simulink model "Project_simulink"  (R2023b)
settings: Solver=VariableStepAuto  StartTime=0.0  StopTime=10.0  RelTol=1e-3
values from neighbouring files (symbols this model uses):
  a = fzero(sun_syncr, R_E)    [project.m]
  A = [A1 A2 A1 A2 A3 A3]    [project.m]
  A_0 = [-cos(phi) -sin(phi) 0; 0 0 1; -sin(phi) cos(phi) 0]    [project.m]
  A_mis_gyros = eye(3) - [0 -mis_gyros(3) mis_gyros(2); mis_gyros(3) 0 -mis_gyros(1); -mis_gyros(2) mis_gyros(1) 0]    [project.m]
  A_mis_MAG = eye(3) - [0 -mis_MAG(3) mis_MAG(2); mis_MAG(3) 0 -mis_MAG(1); -mis_MAG(2) mis_MAG(1) 0]    [project.m]
  a_S = kep_E(1)    [project.m]
  Acc = 0.75e-2    (= 0.0075)    [project.m]
  alpha = 0.9    [plotPlanet.m]    (also in project.m = [alpha_1 alpha_2]')
  alpha_error_slew_min = deg2rad(10)    [project.m]
  alpha_G_0 = deg2rad(0)    [project.m]
  Area_coil = pi * diameter_coil^2/4    (= 0.000706858347058)    [project.m]
  coil_nominal_resistance = max_voltage_torq^2/power_max_coil    (= 81.6666666667)    [project.m]
  DCM_MIS_SS = eye(3) - [0 -mis_ss(3) mis_ss(2); mis_ss(3) 0 -mis_ss(1); -mis_ss(2) mis_ss(1) 0]    [project.m]
  DCM_SS_B = eye(3)    [project.m]
  e = 0    [project.m]
  e_S = kep_E(2)    [project.m]
  f = 15    [project.m]
  f_mag = 5    [project.m]
  FS_mag = 30    [project.m]
  g = [g1_0 g2_0 g3_0 g4_0 g5_0 g6_0 g7_0 g8_0 g9_0 g10_0  g11_0  g12_0  g13_0 ... (first row only)    [IGRF13_2020.m]
  h = [h1_0 h2_0 h3_0 h4_0 h5_0 h6_0 h7_0 h8_0 h9_0 h10_0  h11_0  h12_0  h13_0 ... (first row only)    [IGRF13_2020.m]
  h_max_RW = 25    [project.m]
  I = diag([Ix_b+Ix_s,Iy_b+Iy_s,Iz_b+Iz_s])    [project.m]
  i = deg2rad(98.3)    [project.m]
  i_S = kep_E(3)    [project.m]
  Izz_RW = 1/2*m_RW*(r_RW^2)    (= 0.12168)    [project.m]
  j_b = 1.4e-3 *[0.2 0.2 1]'*m    [project.m]
  K1_slew = 433*[1,1,1]    [project.m]
  K2_slew = 2.19*[1,1,1]    [project.m]
  k_filt_g = 0.75    [project.m]
  k_filt_m = 0.75    [project.m]
  k_filt_s = 0.75    [project.m]
  K_non_lin = 0.1    [project.m]
  Kb = (1e8)    (= 100000000)    [project.m]
  Kdx = 0.5    [project.m]
  Kdy = Kdx    (= 0.5)    [project.m]
  Kdz = 0.5    [project.m]
  Kpx = 0.005    [project.m]
  Kpy = Kpx    (= 0.005)    [project.m]
  Kpz = 0.005    [project.m]
  Lin = 0.015e-2    (= 0.00015)    [project.m]
  linearity_mag_error = 0.02    [project.m]
  max_voltage_torq = 14    [project.m]
  Mounting_error_RW = eye(3) - [0 -mis_RW(3) mis_RW(2); mis_RW(3) 0 -mis_RW(1); -mis_RW(2) mis_RW(1) 0]    [project.m]
  Mounting_matrix_RW = eye(3)    [project.m]
  mu_E = astroConstants(13)    [project.m]
  n = sqrt(mu_E/a^3)    [project.m]
  N_B = [1 0 0; 0 1 0; -1 0 0; 0 -1 0; 0 0 1; 0 0 -1]'    [project.m]
  n_coil = ceil(magnetic_dipole_max/(Area_coil*current_max_coil))    [project.m]
  n_order = 13    [project.m]
  n_S = 2*pi/T_S    [project.m]
  nA_coeff = n_coil*Area_coil    [project.m]
  Noise_Mag = (12e-12)^2    (= 1.44e-22)    [project.m]
  noise_pwm = 50e-6    (= 5e-05)    [project.m]
  Noise_sun_sensor = deg2rad(Acc_ss)^2*t_ss    [project.m]
  OM = deg2rad(270)    [project.m]
  om = 0    [project.m]
  om_0 = [0.08 0.08 0.08]'    [project.m]
  om_detumbling = 4*n    [project.m]
  om_error_slew_min = 0.1*n    [project.m]
  om_target = [0,0,n]'    [project.m]
  P = Fe/c    [project.m]
  r_F = [l1/2 0 0; 0 l2/2 0; -l1/2 0 0; 0 -l2/2 0; 0 0 (l3+l3_s)/2; 0 0 -(l3+l3_s)/2]'    [project.m]
  R_th = 0.1    [project.m]
  residual_dipole = abs(0.005*magnetic_dipole_max*randn)    [project.m]
  resistance_tol = 0.05*randn    [project.m]
  rho_d = 0.1*ones(6,1)    [project.m]
  rho_S = [0.5, 0.5, 0.5, 0.5, 0.5, 0.1]    [project.m]
  RW_axis = [0;0;1]    [project.m]
  sample_time = 1/f    (= 0.0666666666667)    [project.m]
  sample_time_mag = 1/f_mag    (= 0.2)    [project.m]
  Sens = 100e-6/1e-9    (= 100000)    [project.m]
  Sensor_fov_direction = cos(FS/2)    [project.m]
  Sensor_normal_direction = [0 0 -1]'    [project.m]
  SF_a = 30 * 1e-6    (= 3e-05)    [project.m]
  SF_nl = 30 * 1e-6    (= 3e-05)    [project.m]
  SF_r = 30 * 1e-6    (= 3e-05)    [project.m]
  T_RW_max = 0.2    [project.m]
  t_ss = 1/f_ss    (= 0.2)    [project.m]
  TCR = 0.0039    [project.m]
  th0 = 0    [project.m]
  th_0_S = kep_E(6)    [project.m]
  w0_RW = w_max_RW/4    (= 91.6297857297)    [project.m]
  w_max_RW = 3500*(2*pi)/60    (= 366.519142919)    [project.m]
  w_RW_error = h_RW_error/Izz_RW    (= 0.0164365548981)    [project.m]
undefined symbols (not defined in the file or in its folder): A0, DiscIntNeverNeededParam
libraries: matrix_library x18, simulink x4, vrlib x3
(part 1 of 2)
settings Model: Creator=pietr  LastModifiedBy=dav20

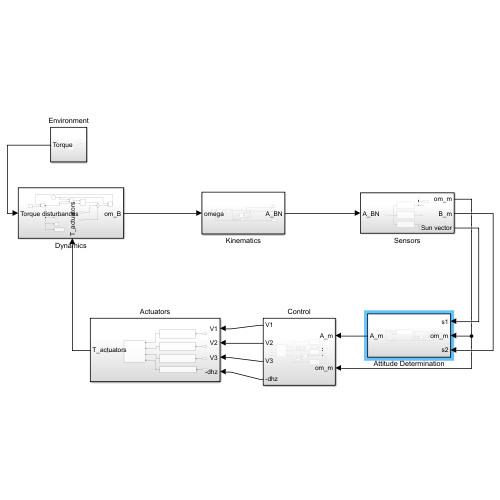
[thumbnail: Simulink's stored preview of the top-level diagram]
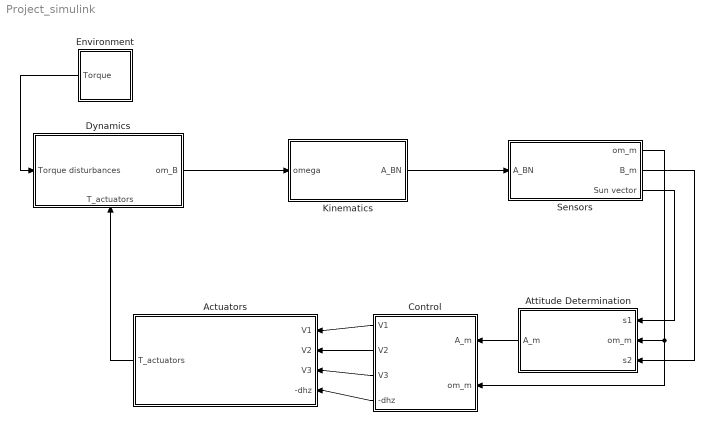
== system Project_simulink ==
  Actuators : Subsystem
  Attitude Determination : Subsystem
  Control : Subsystem
  Dynamics : Subsystem
      settings: PortSchema="{\"entries\":[{\"content\":{\"sides\":[{\"content\":{\"connectorIds\":[\"In1\"]},\"type\":\"ConnectorPlacement.EquallySpacedRectSide\",\"uuid\":\"97ef2013-c355-4554-819d-1d207ceebda7\"},{\"content\":{\"connectorIds\":[\"Out1\"],\"side\":\"RIGHT\"},\"type\":\"ConnectorPlacement.EquallySpacedRectSide\",\"uuid\":\"5691f1bb-9c80-4fa2-8587-6aaeddeffaf6\"},{\"content\":{\"side\":\"TOP\"},\"type\":\"ConnectorPlacement.EquallySpacedRectSide\",\"uuid\":\"3eac2c16-1979-435f-a318-2465fec9d9b3\"},{\"content\":{\"connectorIds\":[\"In2\"],\"side\":\"BOTTOM\"},\"type\":\"ConnectorPlacement.EquallySpacedRectSide\",\"uuid\":\"9d11ba2d-284a-4dde-a2ab-be6ae89ecb98\"}]},\"type\":\"ConnectorPlacement.EquallySpacedConnector\",\"uuid\":\"86d48b44-f40e-4c8e-8b18-c1912efaa89c\"}],\"packageUris\":[\"http://schema.mathworks.com/mf0/Connector/R2020b\"],\"version\":\"1.0\"}"
  Environment : Subsystem
  Kinematics : Subsystem
  Sensors : Subsystem
  wires:
  Control/2(V2) -> Actuators/2(V2)
  Control/3(V3) -> Actuators/3(V3)
  Control/4(-dhz) -> Actuators/4(-dhz)
  Attitude Determination/1(A_m) -> Control/1(A_m)
  Control/1(V1) -> Actuators/1(V1)
  Environment/1(Torque) -> Dynamics/1(Torque disturbances)
  Dynamics/1(om_B) -> Kinematics/1(omega)
  Kinematics/1(A_BN) -> Sensors/1(A_BN)
  Sensors/1(om_m) -> Control/2(om_m), Attitude Determination/2(om_m)
  Sensors/3(Sun vector) -> Attitude Determination/1(s1)
  Sensors/2(B_m) -> Attitude Determination/3(s2)
  Actuators/1(T_actuators) -> Dynamics/2(T_actuators)

== system Project_simulink/Actuators ==
  V1 : Inport
  V2 : Inport  Port=2
  V3 : Inport  Port=3
  -dhz : Inport  Port=4
  Magnetorquers1 : Subsystem
  Magnetorquers2 : Subsystem
  Magnetorquers3 : Subsystem
  Reaction wheel : Subsystem
  control mode torque : Subsystem
  T_actuators : Outport
  wires:
  Magnetorquers2/1(m_y) -> control mode torque/2(m_y)
  Magnetorquers1/1(m_x) -> control mode torque/1(m_x)
  Magnetorquers3/1(m_z) -> control mode torque/3(m_z)
  Reaction wheel/1(T_RW_Z) -> control mode torque/4(T_RW_Z)
  control mode torque/1(T_actuators) -> T_actuators/1
  V1/1 -> Magnetorquers1/1(Magnetorquer command [V])
  V2/1 -> Magnetorquers2/1(Magnetorquer command [V])
  V3/1 -> Magnetorquers3/1(Magnetorquer command [V])
  -dhz/1 -> Reaction wheel/1(Required derivative angular momentum)

== system Project_simulink/Attitude Determination ==
  s1 : Inport
  om_m : Inport  Port=2
  s2 : Inport  Port=3
  "Attitude determination Wabha problem " : Subsystem
  Attitude determination kinematic method : Subsystem
  Dot Product : DotProduct  OutDataTypeStr=Inherit: Inherit via internal rule
  Switch : Switch  Criteria=u2 > Threshold  Threshold=0.5  SaturateOnIntegerOverflow=off  InputSameDT=off
  A_m : Outport
  wires:
  s2/1 -> "Attitude determination Wabha problem "/2(s2)
  [S_N] -> "Attitude determination Wabha problem "/3(v1)
  [B_N] -> "Attitude determination Wabha problem "/4(v2)
  "Attitude determination Wabha problem "/1(A_m_sensor) -> Switch/1, Attitude determination kinematic method/1(A_m)
  om_m/1 -> Attitude determination kinematic method/3(omega)
  Attitude determination kinematic method/1(A_m_gyro) -> Switch/3
  Switch/1 -> A_m/1
  Dot Product/1 -> Attitude determination kinematic method/2(s1_cond), Switch/2  "sun_sensor_condition"
  s1/1 -> Dot Product/2, Dot Product/1, "Attitude determination Wabha problem "/1(s1)

== system Project_simulink/Control ==
  A_m : Inport
  om_m : Inport  Port=2
  3-axis stabilization : Subsystem
  Detumbling : Subsystem
  Flag condition : Subsystem
  Norm : Subsystem
  Slew manouevre : Subsystem
  To Workspace : ToWorkspace  VariableName=flag_det_slew  SampleTime=-1
  To Workspace1 : ToWorkspace  VariableName=flag_slew_nom  SampleTime=-1
  control mode input actuators : Subsystem
  flag_slewtonom : Subsystem
  V1 : Outport
  V2 : Outport  Port=2
  V3 : Outport  Port=3
  -dhz : Outport  Port=4
  tag scope: flag_det_slew=global, flag_slew_nom=global
  wires:
  A_m/1 -> 3-axis stabilization/2(In2), Slew manouevre/2(In2)
  3-axis stabilization/1(V_nominal) -> control mode input actuators/3(V_nominal)
  Norm/1(norm om_m) -> Flag condition/1(norm om_m)
  om_m/1 -> Norm/1(om_m), Detumbling/1(om_m), flag_slewtonom/1(om_m), 3-axis stabilization/1(om_m), Slew manouevre/1(om_m)
  Detumbling/1(V_detumb1) -> control mode input actuators/1(V_detumbling)
  Slew manouevre/1(V_slew_manouevre) -> control mode input actuators/2(V_slew)
  Slew manouevre/2(alpha errors) -> flag_slewtonom/2(alpha errors)
  flag_slewtonom/1(flag_slew_nom) -> [flag_slew_nom], To Workspace1/1
  Flag condition/1(flag) -> To Workspace/1, [flag_det_slew]
  control mode input actuators/1(V1) -> V1/1
  control mode input actuators/2(V2) -> V2/1
  control mode input actuators/3(V3) -> V3/1
  control mode input actuators/4(-dhz) -> -dhz/1

== system Project_simulink/Dynamics ==
  Torque disturbances : Inport
  T_actuators : Inport  Port=2
  Constant5 : Constant  Value=om_0
  Constant7 : Constant  Value=I
  Cross Product : matrix_library/Cross Product
  Integrator : Integrator  InitialConditionSource=external  InitialCondition=om_0
  Product : Product  Multiplication=Matrix(*)
  Product1 : Product  Inputs=/*  Multiplication=Matrix(*)
  Sum : Sum  Inputs=+++
  To Workspace2 : ToWorkspace  VariableName=om_B  SampleTime=-1
  om_B : Outport
  tag scope: om_B=global
  wires:
  Integrator/1 -> To Workspace2/1, [om_B], om_B/1, Cross Product/2, Product/2
  Product/1 -> Cross Product/1
  Constant5/1 -> Integrator/2
  Constant7/1 -> Product/1, Product1/1
  Product1/1 -> Integrator/1
  Cross Product/1 -> Sum/1
  Torque disturbances/1 -> Sum/2
  T_actuators/1 -> Sum/3
  Sum/1 -> Product1/2

== system Project_simulink/Environment ==
  Gravity Gradient Torque : Subsystem
  Magnetic Torque : Subsystem
  Orbit Definition : Subsystem
  SRP : Subsystem
  Sum : Sum
  To Workspace : ToWorkspace  VariableName=GG  SampleTime=-1
  To Workspace1 : ToWorkspace  VariableName=MAG  SampleTime=-1
  To Workspace2 : ToWorkspace  VariableName=SRP  SampleTime=-1
  To Workspace3 : ToWorkspace  VariableName=Torque  SampleTime=-1
  Torque : Outport
  tag scope: theta=global, theta_dot=global
  wires:
  Orbit Definition/3(r_direction) -> Magnetic Torque/2(r_direction)
  Orbit Definition/2(r_magnitude) -> Gravity Gradient Torque/2(r_magnitude), Magnetic Torque/1(r_magnitude)
  [A_BN] -> Magnetic Torque/3(A_BN), SRP/1(A_BN), Orbit Definition/1(A_BN)
  [A_BL] -> Gravity Gradient Torque/1(A_BL)
  Orbit Definition/1(theta) -> [theta]
  Orbit Definition/4(S_N) -> SRP/2(S_N)
  Orbit Definition/5(theta_dot) -> [theta_dot]
  SRP/1(Output1) -> To Workspace2/1
  Gravity Gradient Torque/1(Gravity Gradient Torque) -> Sum/1, To Workspace/1
  Sum/1 -> Torque/1, To Workspace3/1
  Magnetic Torque/1(Mag_Torque) -> Sum/2, To Workspace1/1

== system Project_simulink/Kinematics ==
  omega : Inport
  Antisymmetric matrix of omega : Subsystem
  Matrix A_BN : Subsystem
  Matrix A_LN : Subsystem
  Matrix Multiply : Product  Multiplication=Matrix(*)
  Product1 : Product  Multiplication=Matrix(*)
  To Workspace1 : ToWorkspace  VariableName=om_N  SampleTime=-1
  Transpose : Math  Operator=transpose
  Transpose1 : Math  Operator=transpose
  A_BN : Outport
  tag scope: A_BL=global, A_BN=global, A_LN=global
  wires:
  omega/1 -> Product1/2, Antisymmetric matrix of omega/1(omega)
  Antisymmetric matrix of omega/1(-omega^) -> Matrix A_BN/1(-omega^)
  Matrix A_BN/1(A_BN) -> A_BN/1, [A_BN], Matrix Multiply/1, Transpose1/1
  Matrix A_LN/1(A_LN) -> [A_LN], Transpose/1
  Transpose/1 -> Matrix Multiply/2
  Matrix Multiply/1 -> [A_BL]
  [theta] -> Matrix A_LN/1(theta)
  Product1/1 -> To Workspace1/1
  Transpose1/1 -> Product1/1

== system Project_simulink/Sensors ==
  A_BN : Inport
  Gyro : Subsystem
  Magnetometer : Subsystem
  Sun sensor : Subsystem
  To Workspace : ToWorkspace  VariableName=om_m  SaveFormat=Timeseries  SampleTime=-1
  To Workspace1 : ToWorkspace  VariableName=B_meas  SampleTime=-1
  om_m : Outport
  B_m : Outport  Port=2
  Sun vector : Outport  Port=3
  tag scope: B_m=global
  wires:
  Sun sensor/1(Sun vector measurement) -> Sun vector/1
  Gyro/1(om_m) -> To Workspace/1, om_m/1
  Magnetometer/1(Output) -> [B_m], To Workspace1/1, B_m/1
  A_BN/1 -> Gyro/1(A_BN), Magnetometer/1(A_BN), Sun sensor/1(A_BN)

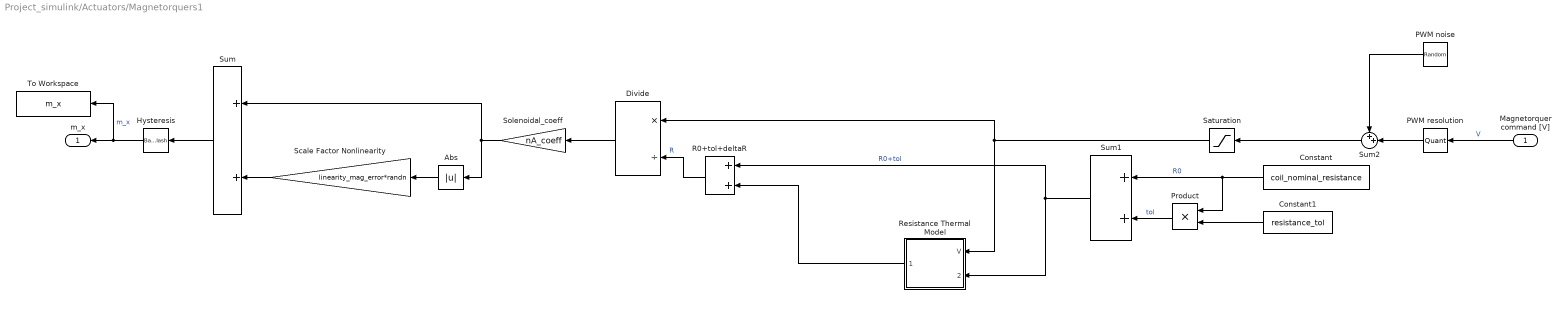
== system Project_simulink/Actuators/Magnetorquers1 ==
  Magnetorquer command [V] : Inport
  Abs : Abs  SaturateOnIntegerOverflow=off
  Constant : Constant  Value=coil_nominal_resistance
  Constant1 : Constant  Value=resistance_tol
  Divide : Product  Inputs=*/
  Hysteresis : Backlash  BacklashWidth=residual_dipole*2
  PWM noise : RandomNumber  Variance=noise_pwm^2  SampleTime=sample_time
  PWM resolution : Quantizer  QuantizationInterval=resolution_pwm
  Product : Product
  R0+tol+deltaR : Sum
  Resistance Thermal Model : Subsystem
  Saturation : Saturate  UpperLimit=max_voltage_torq  LowerLimit=-max_voltage_torq
  Scale Factor Nonlinearity : Gain  Gain=linearity_mag_error*randn
  Solenoidal_coeff : Gain  Gain=nA_coeff
  Sum : Sum
  Sum1 : Sum
  Sum2 : Sum  Inputs=++|
  To Workspace : ToWorkspace  VariableName=m_x  SampleTime=-1
  m_x : Outport
  wires:
  Sum/1 -> Hysteresis/1
  Solenoidal_coeff/1 -> Abs/1, Sum/1
  Scale Factor Nonlinearity/1 -> Sum/2
  Sum1/1 -> Resistance Thermal Model/2(R0+tol), R0+tol+deltaR/1  "R0+tol"
  Constant/1 -> Product/1, Sum1/1  "R0"
  Product/1 -> Sum1/2  "tol"
  Constant1/1 -> Product/2
  Divide/1 -> Solenoidal_coeff/1
  R0+tol+deltaR/1 -> Divide/2  "R"
  Resistance Thermal Model/1(delta R) -> R0+tol+deltaR/2
  Sum2/1 -> Saturation/1
  PWM resolution/1 -> Sum2/2
  PWM noise/1 -> Sum2/1
  Magnetorquer command [V]/1 -> PWM resolution/1  "V"
  Saturation/1 -> Resistance Thermal Model/1(V), Divide/1
  Abs/1 -> Scale Factor Nonlinearity/1
  Hysteresis/1 -> To Workspace/1, m_x/1  "m_x"

== system Project_simulink/Actuators/Magnetorquers2 ==
  Magnetorquer command [V] : Inport
  Abs : Abs  SaturateOnIntegerOverflow=off
  Constant : Constant  Value=coil_nominal_resistance
  Constant1 : Constant  Value=resistance_tol
  Divide : Product  Inputs=*/
  Hysteresis : Backlash  BacklashWidth=residual_dipole*2
  PWM noise : RandomNumber  Variance=noise_pwm^2  SampleTime=sample_time
  PWM resolution : Quantizer  QuantizationInterval=resolution_pwm
  Product : Product
  R0+tol+deltaR : Sum
  Resistance Thermal Model : Subsystem
  Saturation : Saturate  UpperLimit=max_voltage_torq  LowerLimit=-max_voltage_torq
  Scale Factor Nonlinearity : Gain  Gain=linearity_mag_error*randn
  Solenoidal_coeff : Gain  Gain=nA_coeff
  Sum : Sum
  Sum1 : Sum
  Sum2 : Sum  Inputs=++|
  To Workspace : ToWorkspace  VariableName=m_y  SampleTime=-1
  m_y : Outport
  wires:
  Abs/1 -> Scale Factor Nonlinearity/1
  Saturation/1 -> Resistance Thermal Model/1(V), Divide/1
  Magnetorquer command [V]/1 -> PWM resolution/1  "V"
  PWM noise/1 -> Sum2/1
  PWM resolution/1 -> Sum2/2
  Sum2/1 -> Saturation/1
  Resistance Thermal Model/1(delta R) -> R0+tol+deltaR/2
  R0+tol+deltaR/1 -> Divide/2  "R"
  Divide/1 -> Solenoidal_coeff/1
  Constant1/1 -> Product/2
  Product/1 -> Sum1/2  "tol"
  Constant/1 -> Sum1/1, Product/1  "R0"
  Sum1/1 -> Resistance Thermal Model/2(R0+tol), R0+tol+deltaR/1  "R0+tol"
  Scale Factor Nonlinearity/1 -> Sum/2
  Solenoidal_coeff/1 -> Abs/1, Sum/1
  Sum/1 -> Hysteresis/1
  Hysteresis/1 -> To Workspace/1, m_y/1  "m_x"

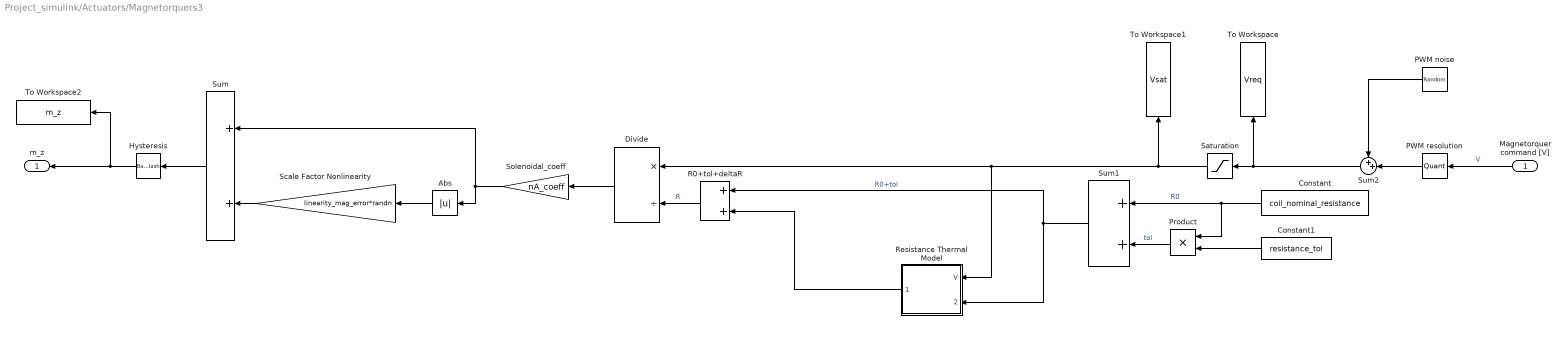
== system Project_simulink/Actuators/Magnetorquers3 ==
  Magnetorquer command [V] : Inport
  Abs : Abs  SaturateOnIntegerOverflow=off
  Constant : Constant  Value=coil_nominal_resistance
  Constant1 : Constant  Value=resistance_tol
  Divide : Product  Inputs=*/
  Hysteresis : Backlash  BacklashWidth=residual_dipole*2
  PWM noise : RandomNumber  Variance=noise_pwm^2  SampleTime=sample_time
  PWM resolution : Quantizer  QuantizationInterval=resolution_pwm
  Product : Product
  R0+tol+deltaR : Sum
  Resistance Thermal Model : Subsystem
  Saturation : Saturate  UpperLimit=max_voltage_torq  LowerLimit=-max_voltage_torq
  Scale Factor Nonlinearity : Gain  Gain=linearity_mag_error*randn
  Solenoidal_coeff : Gain  Gain=nA_coeff
  Sum : Sum
  Sum1 : Sum
  Sum2 : Sum  Inputs=++|
  To Workspace : ToWorkspace  VariableName=Vreq  SampleTime=-1
  To Workspace1 : ToWorkspace  VariableName=Vsat  SampleTime=-1
  To Workspace2 : ToWorkspace  VariableName=m_z  SampleTime=-1
  m_z : Outport
  wires:
  Abs/1 -> Scale Factor Nonlinearity/1
  Saturation/1 -> Resistance Thermal Model/1(V), Divide/1, To Workspace1/1
  Magnetorquer command [V]/1 -> PWM resolution/1  "V"
  PWM noise/1 -> Sum2/1
  PWM resolution/1 -> Sum2/2
  Sum2/1 -> Saturation/1, To Workspace/1
  Resistance Thermal Model/1(delta R) -> R0+tol+deltaR/2
  R0+tol+deltaR/1 -> Divide/2  "R"
  Divide/1 -> Solenoidal_coeff/1
  Constant1/1 -> Product/2
  Product/1 -> Sum1/2  "tol"
  Constant/1 -> Sum1/1, Product/1  "R0"
  Sum1/1 -> Resistance Thermal Model/2(R0+tol), R0+tol+deltaR/1  "R0+tol"
  Scale Factor Nonlinearity/1 -> Sum/2
  Solenoidal_coeff/1 -> Sum/1, Abs/1
  Sum/1 -> Hysteresis/1
  Hysteresis/1 -> To Workspace2/1, m_z/1

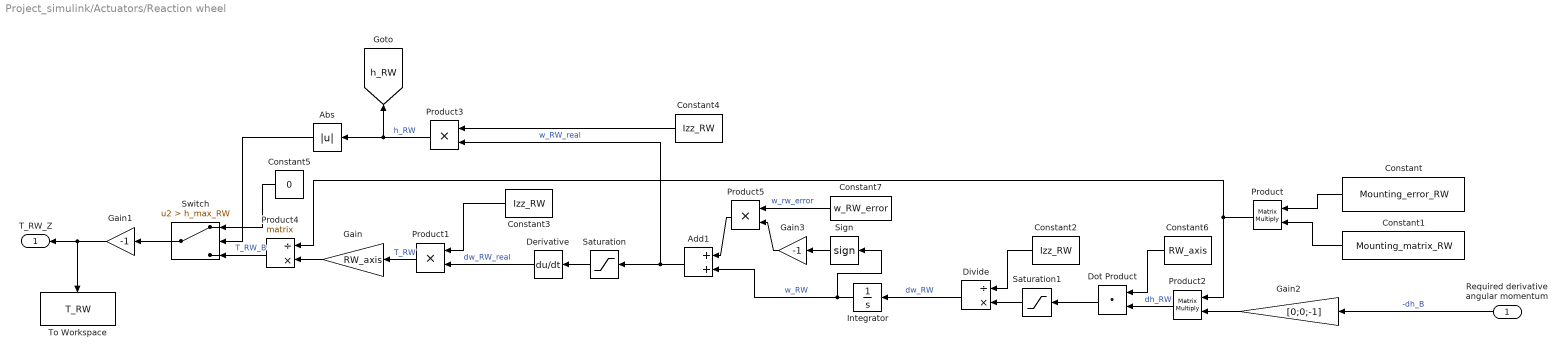
== system Project_simulink/Actuators/Reaction wheel ==
  Required derivative angular momentum : Inport
  Abs : Abs  SaturateOnIntegerOverflow=off
  Add1 : Sum
  Constant : Constant  Value=Mounting_error_RW
  Constant1 : Constant  Value=Mounting_matrix_RW
  Constant2 : Constant  Value=Izz_RW
  Constant3 : Constant  Value=Izz_RW
  Constant4 : Constant  Value=Izz_RW
  Constant5 : Constant  Value=0
  Constant6 : Constant  Value=RW_axis
  Constant7 : Constant  Value=w_RW_error
  Derivative : Derivative
  Divide : Product  Inputs=/*
  Dot Product : DotProduct  OutDataTypeStr=Inherit: Inherit via internal rule
  Gain : Gain  Gain=RW_axis
  Gain1 : Gain  Gain=-1
  Gain2 : Gain  Gain=[0;0;-1]
  Gain3 : Gain  Gain=-1
  Integrator : Integrator  InitialCondition=w0_RW
  Product : Product  Multiplication=Matrix(*)
  Product1 : Product
  Product2 : Product  Multiplication=Matrix(*)
  Product3 : Product
  Product4 : Product  Inputs=/*  Multiplication=Matrix(*)
  Product5 : Product
  Saturation : Saturate  UpperLimit=w_max_RW  LowerLimit=-w_max_RW
  Saturation1 : Saturate  UpperLimit=T_RW_max  LowerLimit=-T_RW_max
  Sign : Signum
  Switch : Switch  Criteria=u2 > Threshold  Threshold=h_max_RW  SaturateOnIntegerOverflow=off  InputSameDT=off
  To Workspace : ToWorkspace  VariableName=T_RW  SampleTime=-1
  T_RW_Z : Outport
  tag scope: h_RW=global
  wires:
  Constant/1 -> Product/1
  Constant1/1 -> Product/2
  Product/1 -> Product2/1, Product4/1
  Required derivative angular momentum/1 -> Gain2/1  "-dh_B"
  Product2/1 -> Dot Product/2  "dh_RW"
  Constant2/1 -> Divide/1
  Divide/1 -> Integrator/1  "dw_RW"
  Integrator/1 -> Sign/1, Add1/2  "w_RW"
  Add1/1 -> Product3/2, Saturation/1  "w_RW_real"
  Saturation/1 -> Derivative/1
  Saturation1/1 -> Divide/2
  Derivative/1 -> Product1/2  "dw_RW_real"
  Constant3/1 -> Product1/1
  Product1/1 -> Gain/1  "T_RW"
  Constant4/1 -> Product3/1
  Product3/1 -> Abs/1, [h_RW]  "h_RW"
  Product4/1 -> Switch/3  "T_RW_B"
  Constant5/1 -> Switch/1
  Abs/1 -> Switch/2
  Dot Product/1 -> Saturation1/1
  Constant6/1 -> Dot Product/1
  Gain/1 -> Product4/2
  Switch/1 -> Gain1/1
  Gain2/1 -> Product2/2
  Sign/1 -> Gain3/1
  Gain3/1 -> Product5/2
  Constant7/1 -> Product5/1  "w_rw_error"
  Product5/1 -> Add1/1
  Gain1/1 -> To Workspace/1, T_RW_Z/1

== system Project_simulink/Actuators/control mode torque ==
  m_x : Inport
  m_y : Inport  Port=2
  m_z : Inport  Port=3
  T_RW_Z : Inport  Port=4
  Subsystem : Subsystem
  Subsystem1 : Subsystem
  Switch : Switch  Threshold=0.5  SaturateOnIntegerOverflow=off  InputSameDT=off
  T_actuators : Outport
  wires:
  m_x/1 -> Subsystem/1(m_x), Subsystem1/1(m_x)
  m_y/1 -> Subsystem/2(m_y), Subsystem1/2(m_y)
  T_RW_Z/1 -> Subsystem/3(T_RW)
  m_z/1 -> Subsystem1/3(m_z)
  [flag_det_slew] -> Switch/2
  Subsystem1/1(T_detumbling) -> Switch/1
  Switch/1 -> T_actuators/1
  Subsystem/1(T_slewornom) -> Switch/3

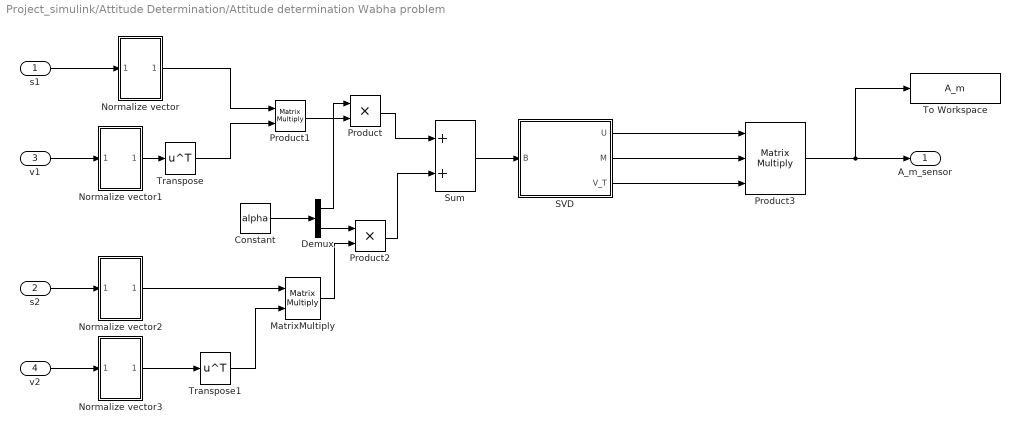
== system Project_simulink/Attitude Determination/Attitude determination Wabha problem  ==
  s1 : Inport
  s2 : Inport  Port=2
  v1 : Inport  Port=3
  v2 : Inport  Port=4
  Constant : Constant  Value=alpha
  Demux : Demux  Outputs=2
  MatrixMultiply : Product  Multiplication=Matrix(*)
  Normalize vector : Subsystem
  Normalize vector1 : Subsystem
  Normalize vector2 : Subsystem
  Normalize vector3 : Subsystem
  Product : Product
  Product1 : Product  Multiplication=Matrix(*)
  Product2 : Product
  Product3 : Product  Inputs=3  Multiplication=Matrix(*)
  SVD : MATLAB Function  TreatAsAtomicUnit=on
  Sum : Sum
  To Workspace : ToWorkspace  VariableName=A_m  SampleTime=-1
  Transpose : Math  Operator=transpose
  Transpose1 : Math  Operator=transpose
  A_m_sensor : Outport
  wires:
  Constant/1 -> Demux/1
  v1/1 -> Normalize vector1/1(In1)
  v2/1 -> Normalize vector3/1(In1)
  Transpose/1 -> Product1/2
  Product1/1 -> Product/2
  Demux/1 -> Product/1
  Transpose1/1 -> MatrixMultiply/2
  s2/1 -> Normalize vector2/1(In1)
  MatrixMultiply/1 -> Product2/2
  Demux/2 -> Product2/1
  Product2/1 -> Sum/2
  Product/1 -> Sum/1
  Sum/1 -> SVD/1(B)
  SVD/1(U) -> Product3/1
  SVD/2(M) -> Product3/2
  SVD/3(V_T) -> Product3/3
  Normalize vector1/1(Out1) -> Transpose/1
  Normalize vector2/1(Out1) -> MatrixMultiply/1
  Normalize vector3/1(Out1) -> Transpose1/1
  Product3/1 -> A_m_sensor/1, To Workspace/1
  s1/1 -> Normalize vector/1(In1)
  Normalize vector/1(Out1) -> Product1/1

== system Project_simulink/Attitude Determination/Attitude determination kinematic method ==
  A_m : Inport
  s1_cond : Inport  Port=2
  omega : Inport  Port=3
  Antisymmetric matrix of omega : Subsystem
  Matrix A_BN : Subsystem
  A_m_gyro : Outport
  wires:
  omega/1 -> Antisymmetric matrix of omega/1(omega)
  Antisymmetric matrix of omega/1(-omega^) -> Matrix A_BN/2(-omega^)
  Matrix A_BN/1(A_m_gyro) -> A_m_gyro/1
  A_m/1 -> Matrix A_BN/3(A_m)
  s1_cond/1 -> Matrix A_BN/1(s1_cond)

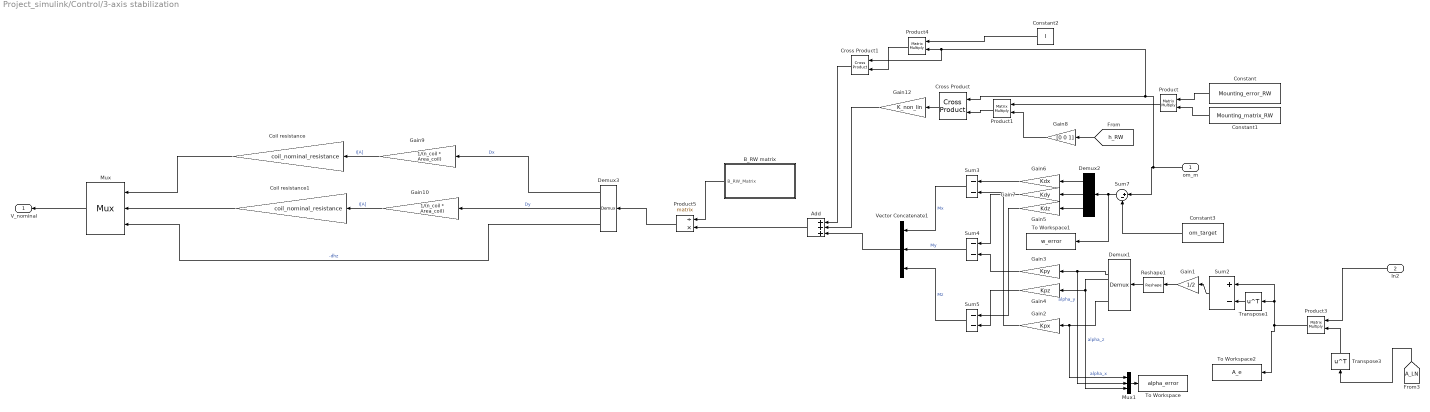
== system Project_simulink/Control/3-axis stabilization ==
  om_m : Inport
  In2 : Inport  Port=2
  Add : Sum  Inputs=+++
  B_RW matrix : Subsystem
  Coil resistance : Gain  Gain=coil_nominal_resistance
  Coil resistance1 : Gain  Gain=coil_nominal_resistance
  Constant : Constant  Value=Mounting_error_RW
  Constant1 : Constant  Value=Mounting_matrix_RW
  Constant2 : Constant  Value=I
  Constant3 : Constant  Value=om_target
  Cross Product : matrix_library/Cross Product
  Cross Product1 : vrlib/Utilities/Cross Product
  Demux1 : Demux  Outputs=9
  Demux2 : Demux  Outputs=3
  Demux3 : Demux  Outputs=3
  Gain1 : Gain  Gain=1/2
  Gain10 : Gain  Gain=1/(n_coil * Area_coil)
  Gain12 : Gain  Gain=K_non_lin
  Gain2 : Gain  Gain=Kpx
  Gain3 : Gain  Gain=Kpy
  Gain4 : Gain  Gain=Kpz
  Gain5 : Gain  Gain=Kdz
  Gain6 : Gain  Gain=Kdx
  Gain7 : Gain  Gain=Kdy
  Gain8 : Gain  Gain=[0 0 1]
  Gain9 : Gain  Gain=1/(n_coil * Area_coil)
  Mux : Mux  Inputs=3
  Mux1 : Mux  Inputs=3
  Product{,1,3..4} (4 alike) : Product  Multiplication=Matrix(*)
  Product5 : Product  Inputs=/*  Multiplication=Matrix(*)
  Reshape1 : Reshape
  Sum2 : Sum  Inputs=+-
  Sum3 : Sum  Inputs=--
  Sum4 : Sum  Inputs=--
  Sum5 : Sum  Inputs=--
  Sum7 : Sum  Inputs=|+-
  To Workspace : ToWorkspace  VariableName=alpha_error  SampleTime=-1
  To Workspace1 : ToWorkspace  VariableName=w_error  SampleTime=-1
  To Workspace2 : ToWorkspace  VariableName=A_e  SampleTime=-1
  Transpose1 : Math  Operator=transpose
  Transpose3 : Math  Operator=transpose
  Vector Concatenate1 : Concatenate  NumInputs=3
  V_nominal : Outport
  wires:
  Sum5/1 -> Vector Concatenate1/3  "Mz"
  om_m/1 -> Sum7/1, Cross Product1/1, Product4/2, Cross Product/1
  Gain2/1 -> Sum3/2
  Gain6/1 -> Sum3/1
  Demux3/2 -> Gain10/1  "Dy"
  Demux1/4 -> Mux1/3, Gain4/1  "alpha_z"
  Demux2/1 -> Gain6/1
  Gain1/1 -> Reshape1/1
  Constant3/1 -> Sum7/2
  Gain3/1 -> Sum4/2
  Product3/1 -> To Workspace2/1, Transpose1/1, Sum2/1
  Demux3/3 -> Mux/3  "-dhz"
  Demux2/3 -> Gain5/1
  Demux1/8 -> Mux1/1, Gain2/1  "alpha_x"
  Sum4/1 -> Vector Concatenate1/2  "My"
  Gain5/1 -> Sum5/1
  Gain10/1 -> Coil resistance1/1  "I[A]"
  Sum7/1 -> To Workspace1/1, Demux2/1
  B_RW matrix/1(B_RW_Matrix) -> Product5/1
  Sum2/1 -> Gain1/1
  Add/1 -> Product5/2
  Sum3/1 -> Vector Concatenate1/1  "Mx"
  Demux1/3 -> Mux1/2, Gain3/1  "alpha_y"
  Demux2/2 -> Gain7/1
  [A_LN] -> Transpose3/1
  Product4/1 -> Cross Product1/2
  Product5/1 -> Demux3/1
  Transpose1/1 -> Sum2/2
  Gain7/1 -> Sum4/1
  Reshape1/1 -> Demux1/1
  Constant2/1 -> Product4/1
  Gain9/1 -> Coil resistance/1  "I[A]"
  Transpose3/1 -> Product3/2
  Gain4/1 -> Sum5/2
  In2/1 -> Product3/1
  Coil resistance/1 -> Mux/1
  Coil resistance1/1 -> Mux/2
  Mux/1 -> V_nominal/1
  Constant/1 -> Product/1
  Constant1/1 -> Product/2
  Product/1 -> Product1/1
  [h_RW] -> Gain8/1
  Vector Concatenate1/1 -> Add/3
  Gain8/1 -> Product1/2
  Cross Product1/1 -> Add/1
  Gain12/1 -> Add/2
  Product1/1 -> Cross Product/2
  Cross Product/1 -> Gain12/1
  Demux3/1 -> Gain9/1  "Dx"
  Mux1/1 -> To Workspace/1

== system Project_simulink/Control/Detumbling ==
  om_m : Inport
  Antisymmetric matrix of omega : Subsystem
  Coil resistance2 : Gain  Gain=coil_nominal_resistance
  Coil resistance3 : Gain  Gain=coil_nominal_resistance
  Coil resistance4 : Gain  Gain=coil_nominal_resistance
  Constant : Constant  Value=Kb
  Demux4 : Demux  Outputs=3
  Gain12 : Gain  Gain=1/(n_coil * Area_coil)
  Gain13 : Gain  Gain=1/(n_coil * Area_coil)
  Gain14 : Gain  Gain=1/(n_coil * Area_coil)
  MatrixMultiply : Product  Multiplication=Matrix(*)
  Mux : Mux  Inputs=3
  Product10 : Product  Inputs=**
  Scope2 : Scope
  To Workspace : ToWorkspace  VariableName=D_desired  SampleTime=-1
  To Workspace1 : ToWorkspace  VariableName=Kb  SampleTime=-1
  V_detumb1 : Outport
  wires:
  Coil resistance4/1 -> Mux/3
  Antisymmetric matrix of omega/1(-omega^) -> MatrixMultiply/1
  Demux4/1 -> Gain14/1  "Dx"
  Demux4/3 -> Gain13/1  "Dz"
  Gain14/1 -> Coil resistance2/1  "I[A]"
  Coil resistance3/1 -> Mux/2
  om_m/1 -> Antisymmetric matrix of omega/1(omega)
  [B_m] -> MatrixMultiply/2
  Gain12/1 -> Coil resistance3/1  "I[A]"
  Gain13/1 -> Coil resistance4/1  "I[A]"
  Demux4/2 -> Gain12/1  "Dy"
  Coil resistance2/1 -> Mux/1
  MatrixMultiply/1 -> Product10/1  "dB"
  Product10/1 -> To Workspace/1, Demux4/1, Scope2/1
  Constant/1 -> Product10/2
  Mux/1 -> V_detumb1/1

== system Project_simulink/Control/Flag condition ==
  norm om_m : Inport
  Clock : Clock
  Constant2 : Constant
  Constant3 : Constant
  Constant4 : Constant  Value=0
  Delay : Delay  DelayLength=1
  Product3 : Product
  Switch : Switch  Criteria=u2 > Threshold  Threshold=om_detumbling  SaturateOnIntegerOverflow=off  InputSameDT=off
  Switch1 : Switch  Threshold=1/f  SaturateOnIntegerOverflow=off  InputSameDT=off
  flag : Outport
  wires:
  Delay/1 -> Switch1/1
  Product3/1 -> flag/1, Delay/1
  Switch1/1 -> Product3/2
  Constant2/1 -> Switch1/3
  Clock/1 -> Switch1/2
  Switch/1 -> Product3/1
  Constant4/1 -> Switch/3
  norm om_m/1 -> Switch/2
  Constant3/1 -> Switch/1

== system Project_simulink/Control/Norm ==
  om_m : Inport
  Dot Product : DotProduct  OutDataTypeStr=Inherit: Inherit via internal rule
  Square Root : Sqrt
  norm om_m : Outport
  wires:
  Square Root/1 -> norm om_m/1
  Dot Product/1 -> Square Root/1
  om_m/1 -> Dot Product/1, Dot Product/2

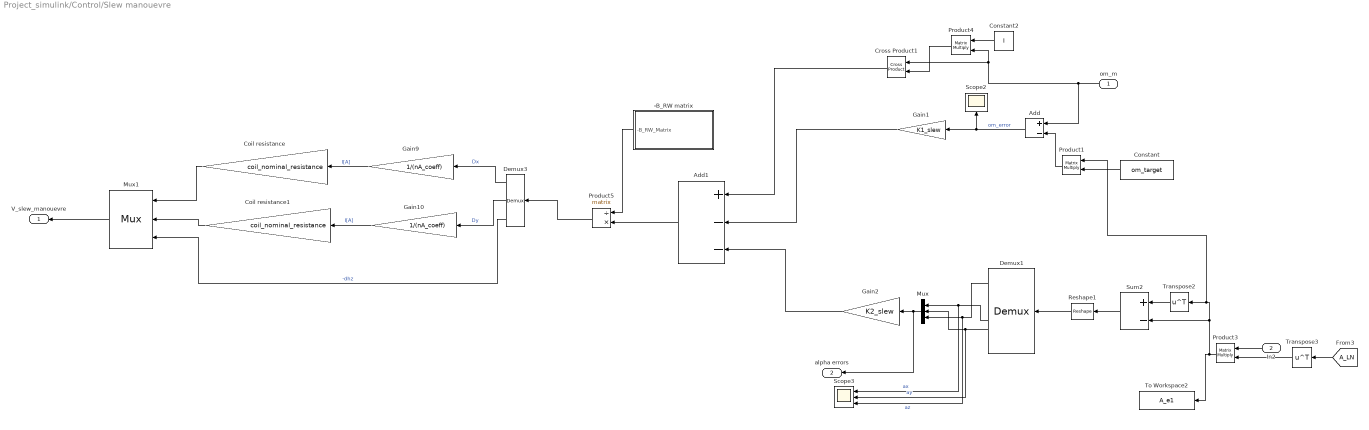
== system Project_simulink/Control/Slew manouevre ==
  om_m : Inport
  In2 : Inport  Port=2
  -B_RW matrix : Subsystem
  Add : Sum  Inputs=+-
  Add1 : Sum  Inputs=+--
  Coil resistance : Gain  Gain=coil_nominal_resistance
  Coil resistance1 : Gain  Gain=coil_nominal_resistance
  Constant : Constant  Value=om_target
  Constant2 : Constant  Value=I
  Cross Product1 : vrlib/Utilities/Cross Product
  Demux1 : Demux  Outputs=9
  Demux3 : Demux  Outputs=3
  Gain1 : Gain  Gain=K1_slew
  Gain10 : Gain  Gain=1/(nA_coeff)
  Gain2 : Gain  Gain=K2_slew
  Gain9 : Gain  Gain=1/(nA_coeff)
  Mux : Mux  Inputs=3
  Mux1 : Mux  Inputs=3
  Product1 : Product  Multiplication=Matrix(*)
  Product3 : Product  Multiplication=Matrix(*)
  Product4 : Product  Multiplication=Matrix(*)
  Product5 : Product  Inputs=/*  Multiplication=Matrix(*)
  Reshape1 : Reshape
  Scope2 : Scope
  Scope3 : Scope  NumInputPorts=3
  Sum2 : Sum  Inputs=+-
  To Workspace2 : ToWorkspace  VariableName=A_e1  SampleTime=-1
  Transpose2 : Math  Operator=transpose
  Transpose3 : Math  Operator=transpose
  V_slew_manouevre : Outport
  alpha errors : Outport  Port=2
  wires:
  Gain1/1 -> Add1/2
  Mux/1 -> alpha errors/1, Gain2/1
  In2/1 -> Product3/1
  Transpose3/1 -> Product3/2
  [A_LN] -> Transpose3/1
  Sum2/1 -> Reshape1/1
  Reshape1/1 -> Demux1/1
  Constant2/1 -> Product4/1
  Product4/1 -> Cross Product1/2
  om_m/1 -> Add/1, Product4/2, Cross Product1/1
  Cross Product1/1 -> Add1/1
  Add/1 -> Scope2/1, Gain1/1  "om_error"
  Gain2/1 -> Add1/3
  Gain9/1 -> Coil resistance/1  "I[A]"
  Coil resistance1/1 -> Mux1/2
  Demux3/1 -> Gain9/1  "Dx"
  -B_RW matrix/1(-B_RW_Matrix) -> Product5/1
  Coil resistance/1 -> Mux1/1
  Product5/1 -> Demux3/1
  Gain10/1 -> Coil resistance1/1  "I[A]"
  Add1/1 -> Product5/2
  Demux3/3 -> Mux1/3  "-dhz"
  Mux1/1 -> V_slew_manouevre/1
  Demux3/2 -> Gain10/1  "Dy"
  Product3/1 -> Sum2/2, Product1/1, Transpose2/1, To Workspace2/1
  Transpose2/1 -> Sum2/1
  Demux1/2 -> Scope3/3, Mux/3  "az"
  Demux1/6 -> Scope3/1, Mux/1  "ax"
  Demux1/7 -> Scope3/2, Mux/2  "ay"
  Constant/1 -> Product1/2
  Product1/1 -> Add/2

== system Project_simulink/Control/control mode input actuators ==
  V_detumbling : Inport
  V_slew : Inport  Port=2
  V_nominal : Inport  Port=3
  Constant : Constant  Value=0
  Demux1 : Demux  Outputs=3
  Switch{1..4} (4 alike) : Switch  Threshold=0.5  SaturateOnIntegerOverflow=off  InputSameDT=off
  V1 : Outport
  V2 : Outport  Port=2
  V3 : Outport  Port=3
  -dhz : Outport  Port=4
  wires:
  Switch2/1 -> Demux1/1
  [flag_det_slew] -> Switch4/2, Switch3/2, Switch2/2
  Demux1/3 -> Switch4/3, Switch3/1
  [flag_slew_nom] -> Switch1/2
  V_nominal/1 -> Switch1/3
  Constant/1 -> Switch3/3, Switch4/1
  V_detumbling/1 -> Switch2/1
  V_slew/1 -> Switch1/1
  Switch1/1 -> Switch2/3
  Demux1/2 -> V2/1
  Demux1/1 -> V1/1
  Switch4/1 -> -dhz/1
  Switch3/1 -> V3/1

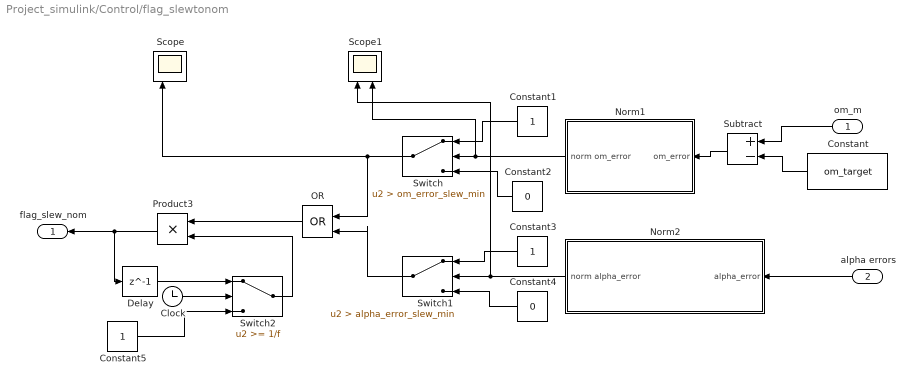
== system Project_simulink/Control/flag_slewtonom ==
  om_m : Inport
  alpha errors : Inport  Port=2
  Clock : Clock
  Constant : Constant  Value=om_target
  Constant1 : Constant
  Constant2 : Constant  Value=0
  Constant3 : Constant
  Constant4 : Constant  Value=0
  Constant5 : Constant
  Delay : Delay  DelayLength=1
  Norm1 : Subsystem
  Norm2 : Subsystem
  OR : Logic  Operator=OR  IconShape=distinctive  AllPortsSameDT=off  OutDataTypeStr=boolean
  Product3 : Product
  Scope : Scope  NumInputPorts=2
  Scope1 : Scope  NumInputPorts=2
  Subtract : Sum  Inputs=+-
  Switch : Switch  Criteria=u2 > Threshold  Threshold=om_error_slew_min  SaturateOnIntegerOverflow=off  InputSameDT=off
  Switch1 : Switch  Criteria=u2 > Threshold  Threshold=alpha_error_slew_min  SaturateOnIntegerOverflow=off  InputSameDT=off
  Switch2 : Switch  Threshold=1/f  SaturateOnIntegerOverflow=off  InputSameDT=off
  flag_slew_nom : Outport
  wires:
  Constant/1 -> Subtract/2
  Norm1/1(norm om_error) -> Scope1/2, Switch/2
  Subtract/1 -> Norm1/1(om_error)
  om_m/1 -> Subtract/1
  alpha errors/1 -> Norm2/1(alpha_error)
  Constant1/1 -> Switch/1
  Constant2/1 -> Switch/3
  Constant4/1 -> Switch1/3
  Constant3/1 -> Switch1/1
  Norm2/1(norm alpha_error) -> Scope1/1, Switch1/2
  Switch/1 -> Scope/1, OR/1
  Product3/1 -> flag_slew_nom/1, Delay/1
  OR/1 -> Product3/1
  Constant5/1 -> Switch2/3
  Clock/1 -> Switch2/2
  Delay/1 -> Switch2/1
  Switch2/1 -> Product3/2
  Switch1/1 -> OR/2

== system Project_simulink/Environment/Gravity Gradient Torque ==
  A_BL : Inport
  r_magnitude : Inport  Port=2
  Constant : Constant  Value=3
  Constant2 : Constant  Value=[1;0;0]
  Constant3 : Constant  Value=I  VectorParams1D=off
  Cross Product : matrix_library/Cross Product
  Divide : Product  Inputs=*/
  Gain : Gain  Gain=3*mu_E
  Gain1 : Gain  Gain=-1
  Matrix Multiply1 : Product  Multiplication=Matrix(*)
  Matrix Multiply2 : Product  Multiplication=Matrix(*)
  Power : Math  Operator=pow
  Gravity Gradient Torque : Outport
  wires:
  Constant3/1 -> Matrix Multiply2/1
  Matrix Multiply1/1 -> Cross Product/2, Matrix Multiply2/2  "[c1; c2; c3]"
  Cross Product/1 -> Gain/1
  Matrix Multiply2/1 -> Cross Product/1
  Constant2/1 -> Matrix Multiply1/2
  A_BL/1 -> Matrix Multiply1/1
  r_magnitude/1 -> Power/1
  Constant/1 -> Power/2
  Power/1 -> Divide/2
  Divide/1 -> Gain1/1
  Gain/1 -> Divide/1
  Gain1/1 -> Gravity Gradient Torque/1

== system Project_simulink/Environment/Magnetic Torque ==
  r_magnitude : Inport
  r_direction : Inport  Port=2
  A_BN : Inport  Port=3
  Clock : Clock
  Constant5 : Constant  Value=j_b
  Constant6 : Constant  Value=g
  Constant7 : Constant  Value=h
  Constant8 : Constant  Value=alpha_G_0
  Constant9 : Constant  Value=n_order
  Cross Product1 : matrix_library/Cross Product
  MATLAB Function : MATLAB Function  TreatAsAtomicUnit=on
  MatrixMultiply : Product  Multiplication=Matrix(*)
  Product3 : Product
  Reshape : Reshape
  Mag_Torque : Outport
  tag scope: B_B=global, B_N=global
  wires:
  Constant8/1 -> MATLAB Function/5(alpha_G_0)
  Constant6/1 -> MATLAB Function/3(g)
  Constant9/1 -> MATLAB Function/6(n_order)
  A_BN/1 -> MatrixMultiply/1
  r_magnitude/1 -> Product3/2
  Constant5/1 -> Cross Product1/1
  MatrixMultiply/1 -> [B_B], Cross Product1/2
  Cross Product1/1 -> Mag_Torque/1
  r_direction/1 -> Product3/1
  Product3/1 -> MATLAB Function/1(r_n)
  Constant7/1 -> MATLAB Function/4(h)
  Clock/1 -> MATLAB Function/2(t)
  MATLAB Function/1(B_N) -> Reshape/1
  Reshape/1 -> MatrixMultiply/2, [B_N]

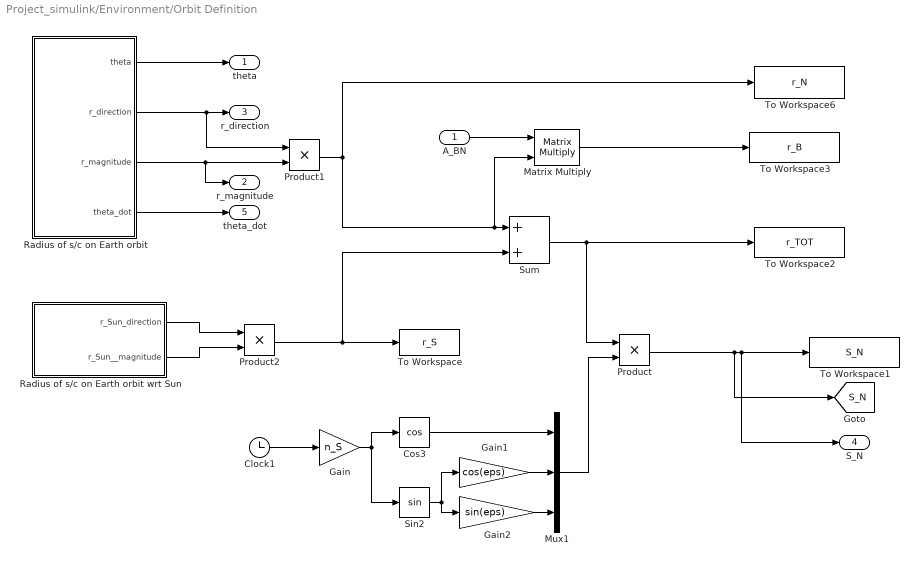
== system Project_simulink/Environment/Orbit Definition ==
  A_BN : Inport
  Clock1 : Clock
  Cos3 : Trigonometry  Operator=cos
  Gain : Gain  Gain=n_S
  Gain1 : Gain  Gain=cos(eps)
  Gain2 : Gain  Gain=sin(eps)
  Matrix Multiply : Product  Multiplication=Matrix(*)
  Mux1 : Mux  Inputs=3
  Product : Product
  Product1 : Product
  Product2 : Product
  Radius of s/c on Earth orbit : Subsystem
  Radius of s/c on Earth orbit wrt Sun : Subsystem
  Sin2 : Trigonometry
  Sum : Sum
  To Workspace : ToWorkspace  VariableName=r_S  SampleTime=-1
  To Workspace1 : ToWorkspace  VariableName=S_N  SampleTime=-1
  To Workspace2 : ToWorkspace  VariableName=r_TOT  SaveFormat=Timeseries  SampleTime=-1
  To Workspace3 : ToWorkspace  VariableName=r_B  SampleTime=-1
  To Workspace6 : ToWorkspace  VariableName=r_N  SampleTime=-1
  theta : Outport
  r_magnitude : Outport  Port=2
  r_direction : Outport  Port=3
  S_N : Outport  Port=4
  theta_dot : Outport  Port=5
  tag scope: S_N=global
  wires:
  Radius of s/c on Earth orbit/1(theta) -> theta/1
  Clock1/1 -> Gain/1
  Sum/1 -> To Workspace2/1, Product/1
  Mux1/1 -> Product/2
  Radius of s/c on Earth orbit/2(r_direction) -> Product1/1, r_direction/1
  Radius of s/c on Earth orbit/3(r_magnitude) -> r_magnitude/1, Product1/2
  Product1/1 -> To Workspace6/1, Matrix Multiply/2, Sum/1
  Radius of s/c on Earth orbit wrt Sun/2(r_Sun__magnitude) -> Product2/2
  Radius of s/c on Earth orbit wrt Sun/1(r_Sun_direction) -> Product2/1
  Product2/1 -> To Workspace/1, Sum/2
  Cos3/1 -> Mux1/1
  Gain/1 -> Sin2/1, Cos3/1
  Sin2/1 -> Gain2/1, Gain1/1
  Gain1/1 -> Mux1/2
  A_BN/1 -> Matrix Multiply/1
  Matrix Multiply/1 -> To Workspace3/1
  Radius of s/c on Earth orbit/4(theta_dot) -> theta_dot/1
  Product/1 -> S_N/1, To Workspace1/1, [S_N]
  Gain2/1 -> Mux1/3

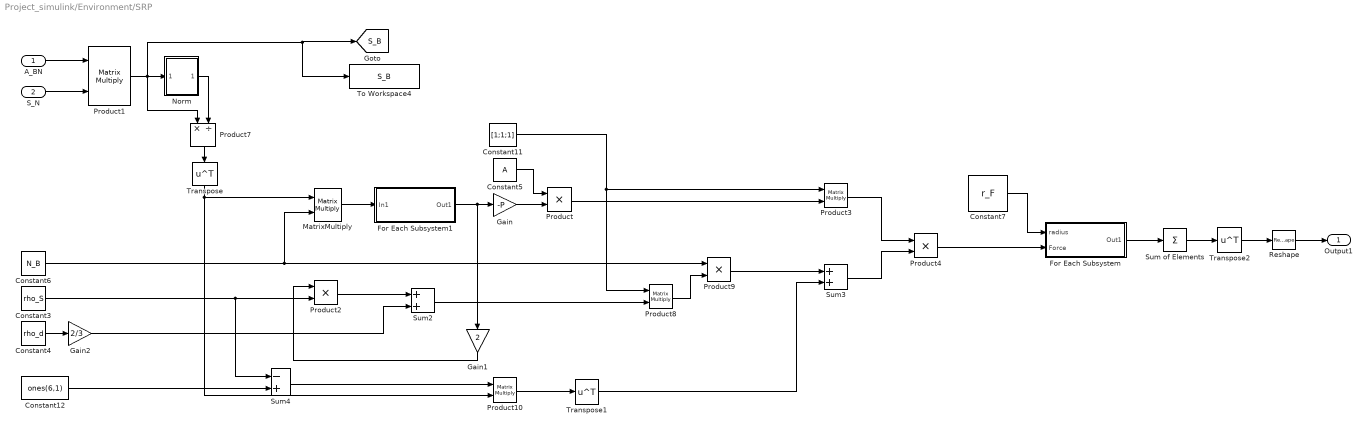
== system Project_simulink/Environment/SRP ==
  A_BN : Inport
  S_N : Inport  Port=2
  Constant11 : Constant  Value=[1;1;1]
  Constant12 : Constant  Value=ones(6,1)
  Constant3 : Constant  Value=rho_S
  Constant4 : Constant  Value=rho_d
  Constant5 : Constant  Value=A
  Constant6 : Constant  Value=N_B
  Constant7 : Constant  Value=r_F
  For Each Subsystem : Subsystem  TreatAsAtomicUnit=on
  For Each Subsystem1 : Subsystem  TreatAsAtomicUnit=on
  Gain : Gain  Gain=-P
  Gain1 : Gain  Gain=2
  Gain2 : Gain  Gain=2/3
  MatrixMultiply : Product  Multiplication=Matrix(*)
  Norm : Subsystem
  Product{,2,4,9} (4 alike) : Product
  Product{1,3,8,10} (4 alike) : Product  Multiplication=Matrix(*)
  Product7 : Product  Inputs=*/
  Reshape : Reshape
  Sum of Elements : Sum  Inputs=+  CollapseMode=Specified dimension  CollapseDim=2
  Sum2 : Sum
  Sum3 : Sum
  Sum4 : Sum  Inputs=-+
  To Workspace4 : ToWorkspace  VariableName=S_B  SampleTime=-1
  Transpose : Math  Operator=transpose
  Transpose1 : Math  Operator=transpose
  Transpose2 : Math  Operator=transpose
  Output1 : Outport
  tag scope: S_B=global
  wires:
  Norm/1(Out1) -> Product7/2
  Product2/1 -> Sum2/1
  Product7/1 -> Transpose/1
  Product1/1 -> [S_B], To Workspace4/1, Norm/1(In1), Product7/1
  Constant4/1 -> Gain2/1
  MatrixMultiply/1 -> For Each Subsystem1/1(In1)
  Sum4/1 -> Product10/1
  Gain/1 -> Product/2
  Constant6/1 -> Product9/1, MatrixMultiply/2
  Gain2/1 -> Sum2/2
  Constant3/1 -> Sum4/1, Product2/2
  Sum of Elements/1 -> Transpose2/1
  Product10/1 -> Transpose1/1
  Product4/1 -> For Each Subsystem/2(Force)
  Gain1/1 -> Product2/1
  Product3/1 -> Product4/1
  Product9/1 -> Sum3/1
  Transpose1/1 -> Sum3/2
  Product8/1 -> Product9/2
  Constant5/1 -> Product/1
  Sum2/1 -> Product8/2
  Transpose/1 -> Product10/2, MatrixMultiply/1
  A_BN/1 -> Product1/1
  Transpose2/1 -> Reshape/1
  Constant7/1 -> For Each Subsystem/1(radius)
  Constant11/1 -> Product8/1, Product3/1
  Product/1 -> Product3/2
  For Each Subsystem/1(Out1) -> Sum of Elements/1
  S_N/1 -> Product1/2
  For Each Subsystem1/1(Out1) -> Gain1/1, Gain/1
  Sum3/1 -> Product4/2
  Reshape/1 -> Output1/1
  Constant12/1 -> Sum4/2

== system Project_simulink/Kinematics/Antisymmetric matrix of omega ==
  omega : Inport
  Constant1 : Constant  Value=[1; 0; 0]  VectorParams1D=off
  Constant2 : Constant  Value=[0; 1; 0]
  Constant3 : Constant  Value=[0; 0; 1]
  Cross Product : matrix_library/Cross Product
  Cross Product1 : matrix_library/Cross Product
  Cross Product2 : matrix_library/Cross Product
  Gain : Gain  Gain=-1
  Mux : Mux  Inputs=3
  Reshape : Reshape  OutputDimensionality=Customize  OutputDimensions=[3,3]
  -omega^ : Outport
  wires:
  omega/1 -> Cross Product/1, Cross Product1/1, Cross Product2/1
  Constant3/1 -> Cross Product2/2
  Cross Product2/1 -> Mux/3
  Cross Product1/1 -> Mux/2
  Mux/1 -> Reshape/1
  Constant2/1 -> Cross Product1/2
  Constant1/1 -> Cross Product/2
  Cross Product/1 -> Mux/1
  Reshape/1 -> Gain/1
  Gain/1 -> -omega^/1

== system Project_simulink/Kinematics/Matrix A_BN ==
  -omega^ : Inport
  Constant5 : Constant  Value=A_0
  Integrator : Integrator  InitialConditionSource=external  InitialCondition=A0
  Orthonormalization of A(t) : Subsystem
  Product : Product  Multiplication=Matrix(*)
  To Workspace : ToWorkspace  VariableName=A_BN  SampleTime=-1
  To Workspace1 : ToWorkspace  VariableName=omega_mat  SampleTime=-1
  A_BN : Outport
  wires:
  Constant5/1 -> Integrator/2
  Orthonormalization of A(t)/1(A(t) orthonormal) -> To Workspace/1, A_BN/1, Product/2  "A_BN"
  Integrator/1 -> Orthonormalization of A(t)/1(A(t))  "A(t)"
  Product/1 -> Integrator/1
  -omega^/1 -> To Workspace1/1, Product/1

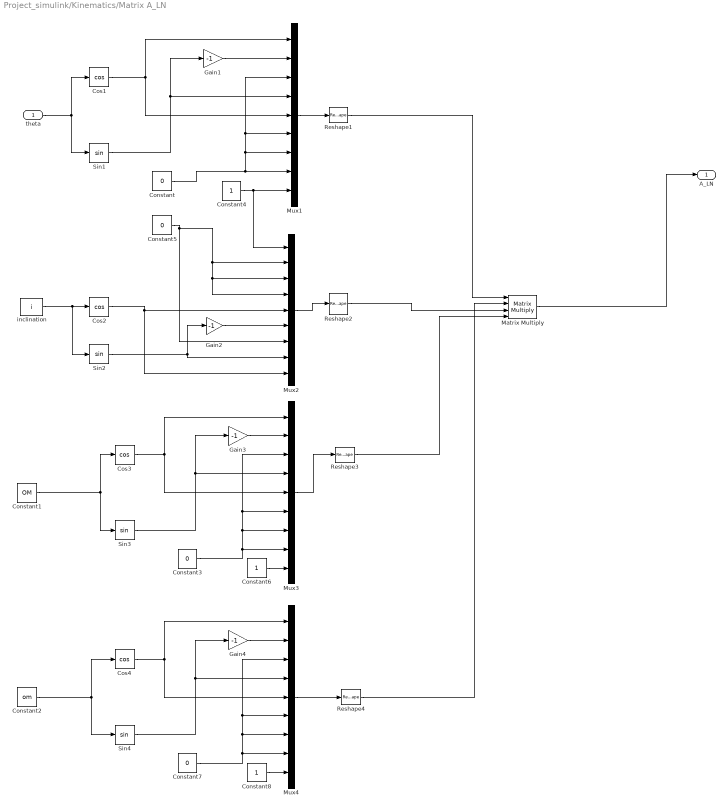
== system Project_simulink/Kinematics/Matrix A_LN ==
  theta : Inport
  Constant{,3,5,7} (4 alike) : Constant  Value=0
  Constant1 : Constant  Value=OM
  Constant2 : Constant  Value=om
  Constant4 : Constant
  Constant6 : Constant
  Constant8 : Constant
  Cos{1..4} (4 alike) : Trigonometry  Operator=cos
  Gain{1..4} (4 alike) : Gain  Gain=-1
  Matrix Multiply : Product  Inputs=4  Multiplication=Matrix(*)
  Mux{1..4} (4 alike) : Mux  Inputs=9
  Reshape{1..4} (4 alike) : Reshape  OutputDimensionality=Customize  OutputDimensions=[3,3]
  Sin{1..4} (4 alike) : Trigonometry
  inclination : Constant  Value=i
  A_LN : Outport
  wires:
  Constant5/1 -> Mux2/4, Mux2/3, Mux2/2, Mux2/7
  Gain2/1 -> Mux2/6
  Constant4/1 -> Mux2/1, Mux1/9
  Sin2/1 -> Gain2/1, Mux2/8
  Cos2/1 -> Mux2/5, Mux2/9
  Gain1/1 -> Mux1/2
  Sin1/1 -> Gain1/1, Mux1/4
  theta/1 -> Cos1/1, Sin1/1
  Constant/1 -> Mux1/8, Mux1/7, Mux1/6, Mux1/3
  Mux2/1 -> Reshape2/1
  inclination/1 -> Sin2/1, Cos2/1
  Mux1/1 -> Reshape1/1
  Cos1/1 -> Mux1/5, Mux1/1
  Cos3/1 -> Mux3/5, Mux3/1
  Constant3/1 -> Mux3/8, Mux3/7, Mux3/6, Mux3/3
  Constant6/1 -> Mux3/9
  Mux3/1 -> Reshape3/1
  Gain3/1 -> Mux3/2
  Constant1/1 -> Sin3/1, Cos3/1
  Sin3/1 -> Gain3/1, Mux3/4
  Cos4/1 -> Mux4/5, Mux4/1
  Constant7/1 -> Mux4/8, Mux4/7, Mux4/6, Mux4/3
  Constant8/1 -> Mux4/9
  Mux4/1 -> Reshape4/1
  Gain4/1 -> Mux4/2
  Constant2/1 -> Sin4/1, Cos4/1
  Sin4/1 -> Gain4/1, Mux4/4
  Matrix Multiply/1 -> A_LN/1
  Reshape1/1 -> Matrix Multiply/1
  Reshape2/1 -> Matrix Multiply/3
  Reshape3/1 -> Matrix Multiply/4
  Reshape4/1 -> Matrix Multiply/2

== system Project_simulink/Sensors/Gyro ==
  A_BN : Inport
  ARW : simulink/Sources/Band-Limited White Noise  Cov=ARW  Ts=sample_time  seed=[23341]
  Abs : Abs  SaturateOnIntegerOverflow=off
  Constant : Constant  Value=A_mis_gyros
  Discrete-Time Integrator1 : DiscreteIntegrator  SampleTime=sample_time  ICPrevOutput=DiscIntNeverNeededParam  ICPrevScaledInput=DiscIntNeverNeededParam
  Filter : Subsystem
  Gain1 : Gain  Gain=SF_r
  Gain2 : Gain  Gain=SF_nl
  Gain3 : Gain  Gain=SF_a
  Product : Product  Multiplication=Matrix(*)
  Quantizer : Quantizer  QuantizationInterval=Resolution
  RRW : simulink/Sources/Band-Limited White Noise  Cov=RRW  Ts=sample_time  seed=[23341]
  Saturation : Saturate  UpperLimit=deg2rad(400)  LowerLimit=deg2rad(-400)
  Square : Math  Operator=square
  Sum : Sum  Inputs=+++
  Sum1 : Sum  Inputs=++++
  Zero-Order Hold : ZeroOrderHold  SampleTime=-1
  om_m : Outport
  wires:
  RRW/1 -> Discrete-Time Integrator1/1
  Quantizer/1 -> Saturation/1
  Sum/1 -> Quantizer/1
  Saturation/1 -> Zero-Order Hold/1
  Square/1 -> Gain2/1
  Gain2/1 -> Sum1/4
  Gain1/1 -> Sum1/2
  Sum1/1 -> Sum/1
  Product/1 -> Abs/1, Square/1, Gain1/1, Sum1/1
  Constant/1 -> Product/1
  Zero-Order Hold/1 -> Filter/1(Input)
  Discrete-Time Integrator1/1 -> Sum/2  "bias"
  ARW/1 -> Sum/3
  Abs/1 -> Gain3/1
  Gain3/1 -> Sum1/3
  Filter/1(Output) -> om_m/1
  [om_B] -> Product/2

== system Project_simulink/Sensors/Magnetometer ==
  A_BN : Inport
  Accuracy : RandomNumber  Variance=(Acc*FS_mag/Sens)^2  SampleTime=1/f_mag
  Band-Limited White Noise : simulink/Sources/Band-Limited White Noise  Cov=[Noise_Mag]  Ts=sample_time_mag  seed=[23341]
  Constant : Constant  Value=A_mis_MAG
  Filter : Subsystem
  Linearity : RandomNumber  Variance=(Lin*FS_mag/Sens)^2  SampleTime=1/f_mag
  Product : Product  Multiplication=Matrix(*)
  Quantizer : Quantizer  QuantizationInterval=Res_mag
  Saturation : Saturate  UpperLimit=1e-4  LowerLimit=-1e-4
  Sum : Sum  Inputs=|++
  Sum1 : Sum  Inputs=+++
  To Workspace2 : ToWorkspace  VariableName=B_m  SampleTime=-1
  Zero-Order Hold : ZeroOrderHold  SampleTime=-1
  Output : Outport
  wires:
  Zero-Order Hold/1 -> Filter/1(Input)
  Accuracy/1 -> Sum1/3
  [B_B] -> Product/2
  Saturation/1 -> Zero-Order Hold/1
  Linearity/1 -> Sum1/2
  Sum1/1 -> Sum/1
  Product/1 -> Sum1/1
  Sum/1 -> Quantizer/1
  Band-Limited White Noise/1 -> Sum/2
  Constant/1 -> Product/1
  Filter/1(Output) -> Output/1, To Workspace2/1
  Quantizer/1 -> Saturation/1

== system Project_simulink/Sensors/Sun sensor ==
  A_BN : Inport
  Band-Limited White Noise1 : simulink/Sources/Band-Limited White Noise  Cov=[Noise_sun_sensor]  Ts=t_ss  seed=[23341]
  Constant : Constant  Value=DCM_MIS_SS
  Constant1 : Constant  Value=DCM_SS_B
  Constant2 : Constant  Value=Sensor_normal_direction
  Constant3 : Constant  Value=[0;0;0]
  Constant4 : Constant  Value=Sensor_fov_direction
  Dot Product : DotProduct  OutDataTypeStr=Inherit: Inherit via internal rule
  Filter : Subsystem
  GreaterThan : RelationalOperator  Operator=>  OutDataTypeStr=boolean  RndMeth=Simplest  InputSameDT=off
  Product : Product  Multiplication=Matrix(*)
  Product1 : Product  Multiplication=Matrix(*)
  Quantizer : Quantizer  QuantizationInterval=res_ss
  Sum : Sum
  Switch : Switch  Criteria=u2 > Threshold  SaturateOnIntegerOverflow=off  InputSameDT=off
  Unit vector : Subsystem
  Zero-Order Hold : ZeroOrderHold  SampleTime=-1
  Sun vector measurement : Outport
  wires:
  Dot Product/1 -> GreaterThan/1
  GreaterThan/1 -> Switch/2
  Quantizer/1 -> Zero-Order Hold/1
  Constant2/1 -> Dot Product/2
  Constant3/1 -> Switch/3
  Band-Limited White Noise1/1 -> Sum/2
  Product/1 -> Product1/1
  Unit vector/1(Out1) -> Product1/2
  Constant1/1 -> Product/2
  Sum/1 -> Quantizer/1
  Constant/1 -> Product/1
  [S_B] -> Unit vector/1(Sun vector)
  Product1/1 -> Sum/1
  Zero-Order Hold/1 -> Dot Product/1, Switch/1
  Constant4/1 -> GreaterThan/2
  Switch/1 -> Filter/1(Input)
  Filter/1(Output) -> Sun vector measurement/1

== system Project_simulink/Actuators/Magnetorquers1/Resistance Thermal Model ==
  V : Inport
  R0+tol : Inport  Port=2
  Constant2 : Constant  Value=R_th
  Constant3 : Constant  Value=TCR
  P=V^2/R : Product  Inputs=*/
  Square1 : Math  Operator=square
  delta R=delta T*TCR : Product
  delta T=P*R_th : Product
  delta R : Outport
  wires:
  R0+tol/1 -> P=V^2/R/2
  delta R=delta T*TCR/1 -> delta R/1
  Constant2/1 -> delta T=P*R_th/1
  delta T=P*R_th/1 -> delta R=delta T*TCR/2
  P=V^2/R/1 -> delta T=P*R_th/2
  V/1 -> Square1/1
  Constant3/1 -> delta R=delta T*TCR/1
  Square1/1 -> P=V^2/R/1

== system Project_simulink/Actuators/Magnetorquers2/Resistance Thermal Model ==
  V : Inport
  R0+tol : Inport  Port=2
  Constant2 : Constant  Value=R_th
  Constant3 : Constant  Value=TCR
  P=V^2/R : Product  Inputs=*/
  Square1 : Math  Operator=square
  delta R=delta T*TCR : Product
  delta T=P*R_th : Product
  delta R : Outport
  wires:
  R0+tol/1 -> P=V^2/R/2
  delta R=delta T*TCR/1 -> delta R/1
  Constant2/1 -> delta T=P*R_th/1
  delta T=P*R_th/1 -> delta R=delta T*TCR/2
  P=V^2/R/1 -> delta T=P*R_th/2
  V/1 -> Square1/1
  Constant3/1 -> delta R=delta T*TCR/1
  Square1/1 -> P=V^2/R/1

== system Project_simulink/Actuators/Magnetorquers3/Resistance Thermal Model ==
  V : Inport
  R0+tol : Inport  Port=2
  Constant2 : Constant  Value=R_th
  Constant3 : Constant  Value=TCR
  P=V^2/R : Product  Inputs=*/
  Square1 : Math  Operator=square
  delta R=delta T*TCR : Product
  delta T=P*R_th : Product
  delta R : Outport
  wires:
  R0+tol/1 -> P=V^2/R/2
  delta R=delta T*TCR/1 -> delta R/1
  Constant2/1 -> delta T=P*R_th/1
  delta T=P*R_th/1 -> delta R=delta T*TCR/2
  P=V^2/R/1 -> delta T=P*R_th/2
  V/1 -> Square1/1
  Constant3/1 -> delta R=delta T*TCR/1
  Square1/1 -> P=V^2/R/1

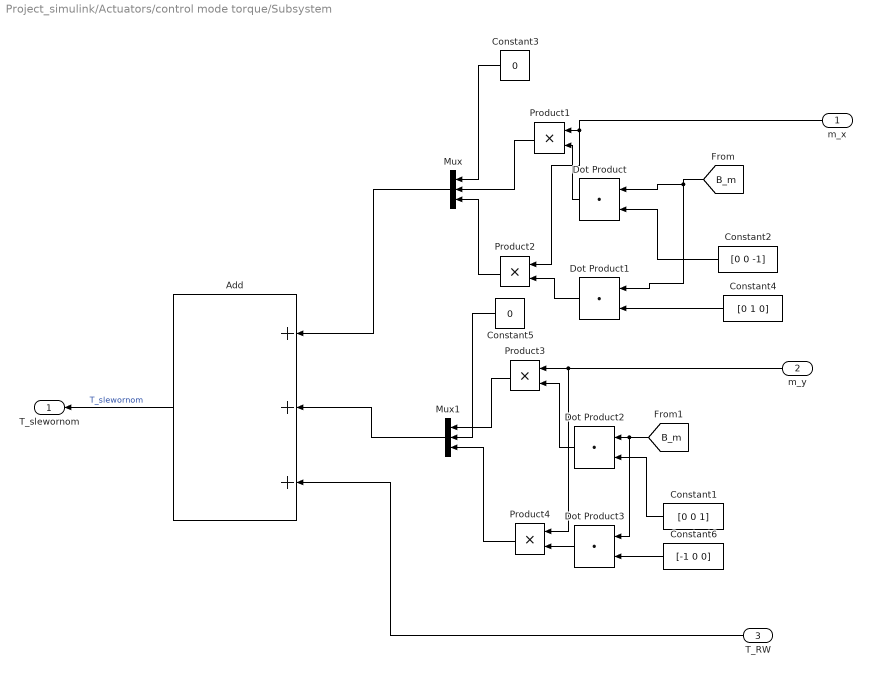
== system Project_simulink/Actuators/control mode torque/Subsystem ==
  m_x : Inport
  m_y : Inport  Port=2
  T_RW : Inport  Port=3
  Add : Sum  Inputs=+++
  Constant1 : Constant  Value=[0 0 1]
  Constant2 : Constant  Value=[0 0 -1]
  Constant3 : Constant  Value=0
  Constant4 : Constant  Value=[0 1 0]
  Constant5 : Constant  Value=0
  Constant6 : Constant  Value=[-1 0 0]
  Dot Product{,1..3} (4 alike) : DotProduct  OutDataTypeStr=Inherit: Inherit via internal rule
  Mux : Mux  Inputs=3
  Mux1 : Mux  Inputs=3
  Product{1..4} (4 alike) : Product
  T_slewornom : Outport
  wires:
  Constant3/1 -> Mux/1
  Product2/1 -> Mux/3
  Dot Product/1 -> Product1/2
  Product3/1 -> Mux1/1
  [B_m] -> Dot Product1/1, Dot Product/1
  m_x/1 -> Product2/1, Product1/1
  Mux/1 -> Add/1
  Constant2/1 -> Dot Product/2
  m_y/1 -> Product4/1, Product3/1
  Dot Product3/1 -> Product4/2
  Constant4/1 -> Dot Product1/2
  Add/1 -> T_slewornom/1  "T_slewornom"
  [B_m] -> Dot Product3/1, Dot Product2/1
  T_RW/1 -> Add/3
  Product1/1 -> Mux/2
  Dot Product1/1 -> Product2/2
  Constant6/1 -> Dot Product3/2
  Dot Product2/1 -> Product3/2
  Constant1/1 -> Dot Product2/2
  Product4/1 -> Mux1/3
  Constant5/1 -> Mux1/2
  Mux1/1 -> Add/2

== system Project_simulink/Actuators/control mode torque/Subsystem1 ==
  m_x : Inport
  m_y : Inport  Port=2
  m_z : Inport  Port=3
  Cross Product : matrix_library/Cross Product
  Mux : Mux  Inputs=3
  T_detumbling : Outport
  wires:
  m_x/1 -> Mux/1
  m_y/1 -> Mux/2
  [B_m] -> Cross Product/2
  Mux/1 -> Cross Product/1
  Cross Product/1 -> T_detumbling/1  "T_detumbling"
  m_z/1 -> Mux/3

== system Project_simulink/Attitude Determination/Attitude determination Wabha problem /Normalize vector ==
  In1 : Inport
  Constant : Constant
  Dot Product : DotProduct  OutDataTypeStr=Inherit: Inherit via internal rule
  Product : Product  Inputs=*/
  Square Root : Sqrt
  Switch : Switch  Criteria=u2 > Threshold  Threshold=0.5  SaturateOnIntegerOverflow=off  InputSameDT=off
  Out1 : Outport
  wires:
  In1/1 -> Product/1, Dot Product/2, Dot Product/1
  Square Root/1 -> Product/2
  Product/1 -> Out1/1
  Dot Product/1 -> Switch/2, Switch/1
  Switch/1 -> Square Root/1
  Constant/1 -> Switch/3
